simulink subsystem "openloop_steering_subsystem"  (R2025b)
settings: Solver=VariableStepAuto  StartTime=0.0  StopTime=10.0  RelTol=1e-3
libraries: simulink x1
settings Model: Creator=orang  LastModifiedBy=erik

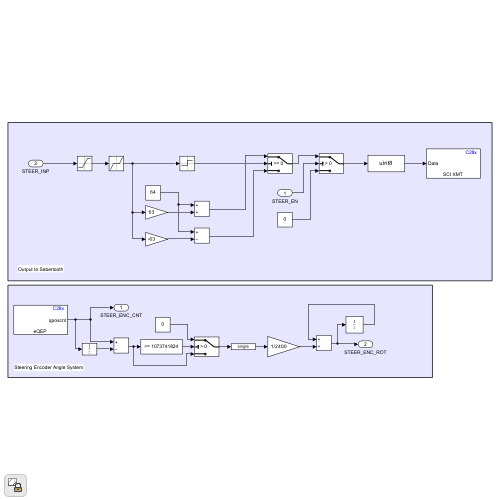
[thumbnail: Simulink's stored preview of the top-level diagram]
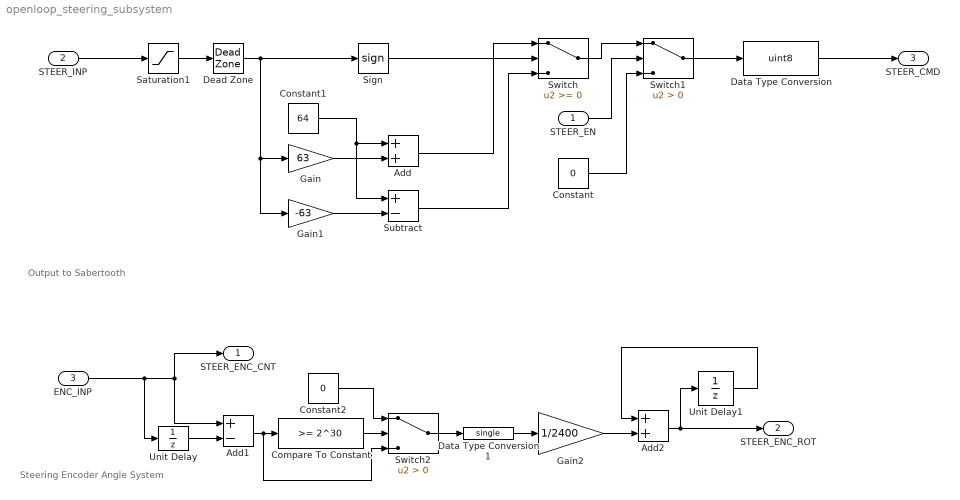
== system openloop_steering_subsystem ==
  note: Steering Encoder Angle System
  note: Output to Sabertooth
  STEER_EN : Inport  OutDataTypeStr=boolean
  STEER_INP : Inport  Port=2
  ENC_INP : Inport  Port=3
  Add : Sum
  Add1 : Sum  Inputs=+-  OutDataTypeStr=int32
  Add2 : Sum
  Compare To Constant : simulink/Logic and Bit Operations/Compare To Constant  relop=>=  const=2^30  OutDataTypeStr=boolean
  Constant : Constant  Value=0
  Constant1 : Constant  Value=64
  Constant2 : Constant  Value=0
  Data Type Conversion : DataTypeConversion  OutDataTypeStr=uint8  SaturateOnIntegerOverflow=off  RndMeth=Floor
  Data Type Conversion1 : DataTypeConversion  OutDataTypeStr=single  SaturateOnIntegerOverflow=off  RndMeth=Floor
  Dead Zone : DeadZone  LowerValue=-0.02  UpperValue=0.02
  Gain : Gain  Gain=63
  Gain1 : Gain  Gain=-63
  Gain2 : Gain  Gain=1/2400
  Saturation1 : Saturate  UpperLimit=1  LowerLimit=-1
  Sign : Signum
  Subtract : Sum  Inputs=+-
  Switch : Switch  SaturateOnIntegerOverflow=off  InputSameDT=off
  Switch1 : Switch  Criteria=u2 > Threshold  SaturateOnIntegerOverflow=off  InputSameDT=off
  Switch2 : Switch  Criteria=u2 > Threshold  SaturateOnIntegerOverflow=off  InputSameDT=off
  Unit Delay : UnitDelay  SampleTime=-1  HasFrameUpgradeWarning=on
  Unit Delay1 : UnitDelay  SampleTime=-1  HasFrameUpgradeWarning=on
  STEER_ENC_CNT : Outport
  STEER_ENC_ROT : Outport  Port=2
  STEER_CMD : Outport  Port=3
  wires:
  Constant/1 -> Switch1/3
  Sign/1 -> Switch/2
  Switch1/1 -> Data Type Conversion/1
  Dead Zone/1 -> Gain/1, Gain1/1, Sign/1
  STEER_EN/1 -> Switch1/2
  Add/1 -> Switch/1
  Data Type Conversion/1 -> STEER_CMD/1
  Constant1/1 -> Add/1, Subtract/1
  Gain/1 -> Add/2
  Gain1/1 -> Subtract/2
  Saturation1/1 -> Dead Zone/1
  Switch/1 -> Switch1/1
  Subtract/1 -> Switch/3
  STEER_INP/1 -> Saturation1/1
  ENC_INP/1 -> Unit Delay/1, STEER_ENC_CNT/1, Add1/1
  Unit Delay/1 -> Add1/2
  Gain2/1 -> Add2/2
  Add2/1 -> Unit Delay1/1, STEER_ENC_ROT/1
  Unit Delay1/1 -> Add2/1
  Data Type Conversion1/1 -> Gain2/1
  Add1/1 -> Compare To Constant/1, Switch2/3
  Switch2/1 -> Data Type Conversion1/1
  Compare To Constant/1 -> Switch2/2
  Constant2/1 -> Switch2/1
